simulink model "testing_time_net_2layers_attempt_2"  (R2018b)
settings: Solver=VariableStepAuto  StartTime=0.0  StopTime=10.0  RelTol=1e-3
values from neighbouring files (symbols this model uses):
  in1 = rand(1,10)'*10    [main_sim_nn.m]
settings Model: Creator=kekatos  LastModifiedBy=kekatos

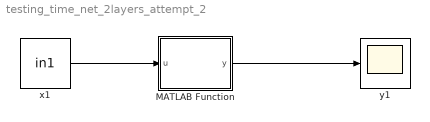
== system testing_time_net_2layers_attempt_2 ==
  MATLAB Function : MATLAB Function  TreatAsAtomicUnit=on
  x1 : Constant  Value=in1  SampleTime=1
      mask Display: e = 0.06;c1 = [120 230 180]/255;c2 = ([120 230 180]+0)/(256+128);c3 = ([120 230 180]+128)/(256+128);patch([0 1 1 0],[0 0 1 1],c1);patch([0 1 1 1-e 1-e 0+e],[0 0 1 1-e 0+e 0+e],c2);patch([0 0 1 1-e 0+e 0+e],[0 1 1 1-e 1-e 0+e],c3);plot([0 1 1 0 0],[0 0 1 1 0]);disp('Constant');
  y1 : Scope
      mask Display: e = 0.06;c1 = [120 230 180]/255;c2 = ([120 230 180]+0)/(256+128);c3 = ([120 230 180]+128)/(256+128);patch([0 1 1 0],[0 0 1 1],c1);patch([0 1 1 1-e 1-e 0+e],[0 0 1 1-e 0+e 0+e],c2);patch([0 0 1 1-e 0+e 0+e],[0 1 1 1-e 1-e 0+e],c3);plot([0 1 1 0 0],[0 0 1 1 0]);plot([0.15 0.85 0.85 0.15 0.15],[0.5 0.5 0.85 0.85 0.5]);
  wires:
  x1/1 -> MATLAB Function/1(u)
  MATLAB Function/1(y) -> y1/1

== matlab function testing_time_net_2layers_attempt_2/MATLAB Function ==
  data: u input; y output; net parameter
function y = fcn(u, net)

global net
% persistent net
% data store memory and parameter
y = sim(net,u);
